simulink model "i2s_mclk_gen"  (R2014b)
settings: Solver=ode45  StartTime=0.0  StopTime=800e-8  RelTol=1e-3
libraries: simulink x1, dspswit3 x1
settings Model: Creator=zhangxin  LastModifiedBy=zhangxin

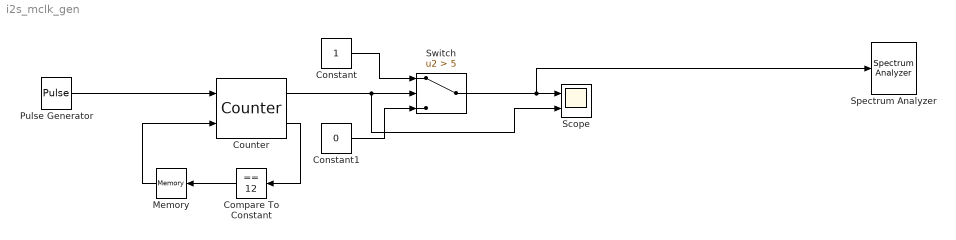
== system i2s_mclk_gen ==
  Compare To Constant : simulink/Logic and Bit Operations/Compare To Constant  relop===  const=12  OutDataTypeStr=boolean
  Constant : Constant
  Constant1 : Constant  Value=0
  Counter : dspswit3/Counter  Direction=Up  CountEvent=Rising edge  CounterSize=8 bits  MaxCount=11  InitialCount=0  Output=Count and Hit  HitValue=12  ResetInput=on  SamplesPerFrame=1  Ts=1  CntDtype=uint8  HitDtype=Logical
  Memory : Memory
  Pulse Generator : DiscretePulseGenerator  PulseType=Time based  Period=1/148.5e6  PulseWidth=50
  Scope : Scope  NumInputPorts=2
      settings: YMin=-5~-5  YMax=5~5
  Spectrum Analyzer : SpectrumAnalyzer
  Switch : Switch  Criteria=u2 > Threshold  Threshold=5  SampleTime=1/148.5e6/2
  wires:
  Pulse Generator/1 -> Counter/1
  Counter/2 -> Compare To Constant/1
  Compare To Constant/1 -> Memory/1
  Memory/1 -> Counter/2
  Counter/1 -> Scope/2, Switch/2
  Constant/1 -> Switch/1
  Constant1/1 -> Switch/3
  Switch/1 -> Spectrum Analyzer/1, Scope/1
